simulink model "NeuralNetUnitLDC_IO"  (R2018b)
settings: Solver=FixedStepAuto  StartTime=0.0  StopTime=20  FixedStep=0.05  RelTol=1e-3
values from neighbouring files (symbols this model uses):
  B = 0.5    [Matlab_Newton_simulation_v01.m]    (also in NewtonMethod.m; NewtonMethod_2.m = 0.3; System_parameters.m = 0.3)
  b = f    (= 0.01)    [Matlab_Newton_simulation_v01.m]    (also in NN_generate_input_data.m = f; NewtonMethod.m; System_parameters.m)
  l = 0.1    [Matlab_Newton_simulation_v01.m]    (also in NewtonMethod.m; NewtonMethod_2.m; System_parameters.m)
  m = 0.04    [Matlab_Newton_simulation_v01.m]    (also in NewtonMethod.m = 0.1; NewtonMethod_2.m; System_parameters.m)
  R = 1    [Matlab_Newton_simulation_v01.m]    (also in NewtonMethod.m; NewtonMethod_2.m = 0.1; System_parameters.m = 0.1)
settings Model: Creator=Therecia  LastModifiedBy=Tyson
settings DebuggingCC: InheritedTsInSrcMsg=none  LibraryContextMissingDiagnostic=none
settings SFSimCC: SimUseLocalCustomCode=off
settings RTWCC: RTWUseLocalCustomCode=off
settings CodeAppCC: StateflowObjectComments=on

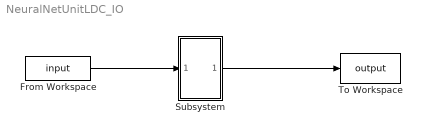
== system NeuralNetUnitLDC_IO ==
  From Workspace : FromWorkspace  VariableName=input
  Subsystem : Subsystem
      mask DialogControl Control2 Prompt: BlackBox
  To Workspace : ToWorkspace  VariableName=output  SaveFormat=Timeseries  SampleTime=-1
  wires:
  From Workspace/1 -> Subsystem/1(In1)
  Subsystem/1(Out1) -> To Workspace/1

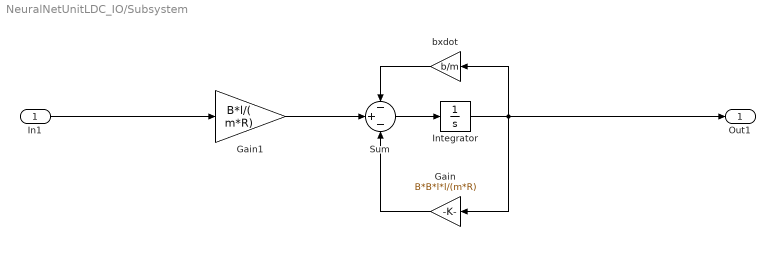
== system NeuralNetUnitLDC_IO/Subsystem ==
  In1 : Inport
  Gain : Gain  Gain=B*B*l*l/(m*R)
  Gain1 : Gain  Gain=B*l/( m*R)
  Integrator : Integrator
  Sum : Sum  Inputs=-+-
  bxdot : Gain  Gain=b/m
  Out1 : Outport
  wires:
  Sum/1 -> Integrator/1
  Gain/1 -> Sum/3
  Gain1/1 -> Sum/2
  bxdot/1 -> Sum/1
  Integrator/1 -> Out1/1, bxdot/1, Gain/1
  In1/1 -> Gain1/1
